simulink model "week2_pr4"  (R2020b)
settings: Solver=VariableStepAuto  StartTime=0.0  StopTime=10.0  RelTol=1e-3
model workspace (MAT data in the model file):
  Var = 0
values from neighbouring files (symbols this model uses):
  b = 3.5076999999999995E-6    [week2_pr4.sldd]
  J = 3.2284E-6    [week2_pr4.sldd]
  K = 0.0274    [week2_pr4.sldd]
  Kd = 0.32314    [week2_pr4.sldd]
  Ki = 1823.1171    [week2_pr4.sldd]
  Kp = 48.9643    [week2_pr4.sldd]
  L = 2.75E-6    [week2_pr4.sldd]
  N = 79169.4921    [week2_pr4.sldd]
  R = 4.0    [week2_pr4.sldd]
settings Model: DataDictionary=week2_pr4.sldd  Creator=user  LastModifiedBy=user

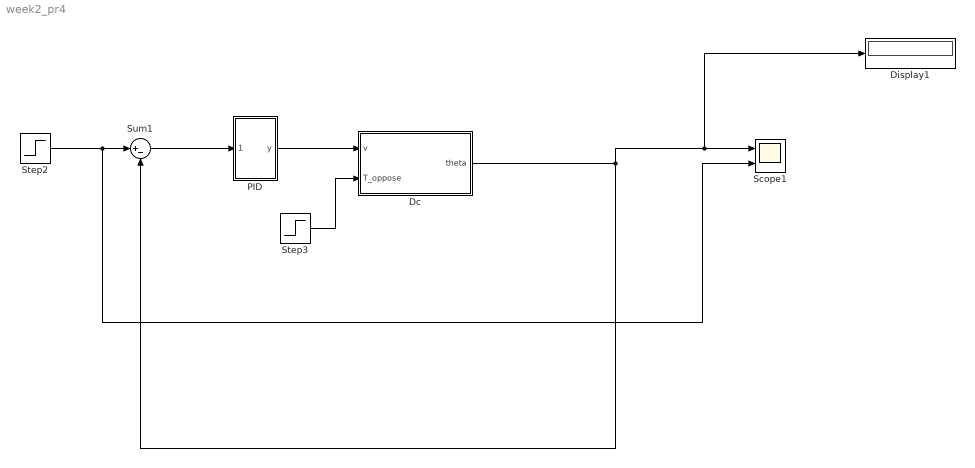
== system week2_pr4 ==
  Dc : Subsystem  TreatAsAtomicUnit=on
  Display1 : Display
  PID : Subsystem  TreatAsAtomicUnit=on
  Scope1 : Scope  NumInputPorts=2
  Step2 : Step  SampleTime=0
  Step3 : Step  SampleTime=0
  Sum1 : Sum  Inputs=|+-
  wires:
  Sum1/1 -> PID/1(error)
  Dc/1(theta) -> Sum1/2, Display1/1, Scope1/1
  Step2/1 -> Scope1/2, Sum1/1
  Step3/1 -> Dc/2(T_oppose)
  PID/1(y) -> Dc/1(v)

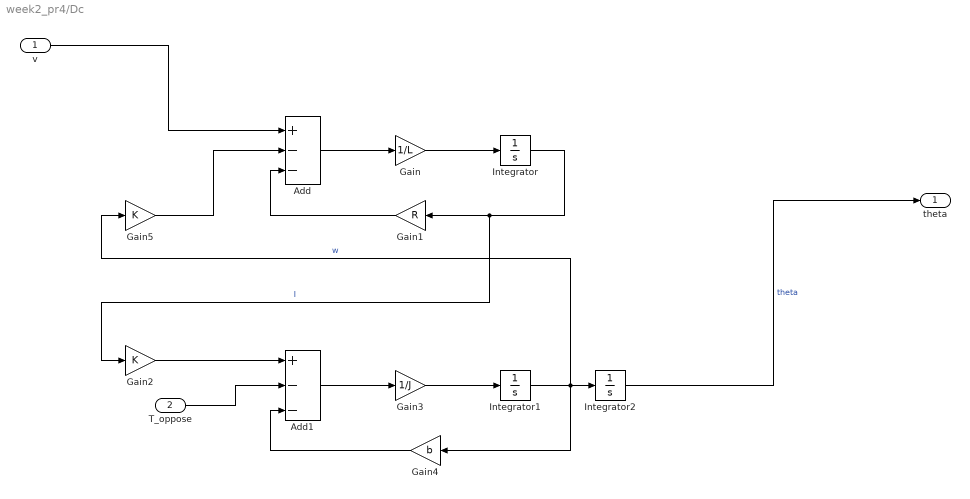
== system week2_pr4/Dc ==
  v : Inport  OutDataTypeStr=double  PortDimensions=1  SampleTime=0
  T_oppose : Inport  Port=2  OutDataTypeStr=double  PortDimensions=1
  Add : Sum  Inputs=+--
  Add1 : Sum  Inputs=+--
  Gain : Gain  Gain=1/L
  Gain1 : Gain  Gain=R
  Gain2 : Gain  Gain=K
  Gain3 : Gain  Gain=1/J
  Gain4 : Gain  Gain=b
  Gain5 : Gain  Gain=K
  Integrator : Integrator
  Integrator1 : Integrator
  Integrator2 : Integrator
  theta : Outport  OutDataTypeStr=double  PortDimensions=1  SampleTime=0
  wires:
  Gain1/1 -> Add/3
  Gain/1 -> Integrator/1
  Add1/1 -> Gain3/1
  Gain3/1 -> Integrator1/1
  Gain5/1 -> Add/2
  Gain4/1 -> Add1/3
  Add/1 -> Gain/1
  Integrator2/1 -> theta/1  "theta"
  T_oppose/1 -> Add1/2
  Integrator/1 -> Gain1/1, Gain2/1  "I"
  Gain2/1 -> Add1/1
  Integrator1/1 -> Integrator2/1, Gain5/1, Gain4/1  "w"
  v/1 -> Add/1

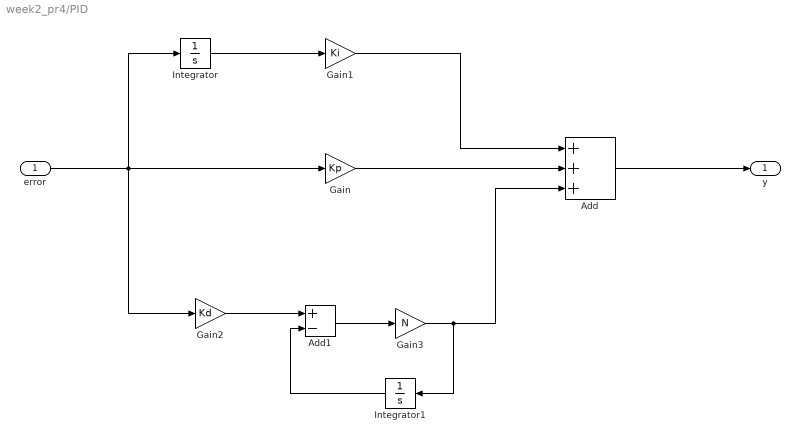
== system week2_pr4/PID ==
  error : Inport  OutDataTypeStr=double  PortDimensions=1  SampleTime=0
  Add : Sum  Inputs=+++
  Add1 : Sum  Inputs=+-
  Gain : Gain  Gain=Kp
  Gain1 : Gain  Gain=Ki
  Gain2 : Gain  Gain=Kd
  Gain3 : Gain  Gain=N
  Integrator : Integrator
  Integrator1 : Integrator
  y : Outport  OutDataTypeStr=double  PortDimensions=1  SampleTime=0
  wires:
  Gain3/1 -> Integrator1/1, Add/3
  Add1/1 -> Gain3/1
  error/1 -> Gain2/1, Gain/1, Integrator/1
  Add/1 -> y/1
  Gain2/1 -> Add1/1
  Integrator/1 -> Gain1/1
  Gain1/1 -> Add/1
  Gain/1 -> Add/2
  Integrator1/1 -> Add1/2
